simulink model "Esercitazione__2"  (R2023b)
settings: Solver=VariableStepAuto  StartTime=0.0  StopTime=10.0  RelTol=1e-3
values from neighbouring files (symbols this model uses):
  CLi = CLvec(j)    [es2.m]    (also in es2_deflussaggio.m)
  Vaprime = Vavec(i)    [es2.m]    (also in es2_deflussaggio.m = 1)
  Vfprime = 1    [es2.m]    (also in es2_deflussaggio.m = bvec(i))
undefined symbols (not defined in the file or in its folder): kteta, kw, taua, Te, Tm, Tteta
settings Model: Creator=marco  LastModifiedBy=39327

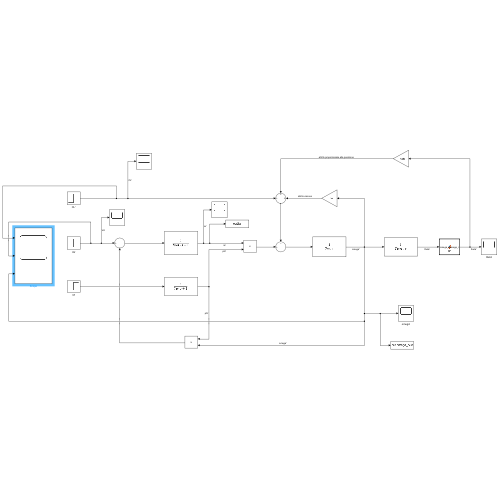
[thumbnail: Simulink's stored preview of the top-level diagram]
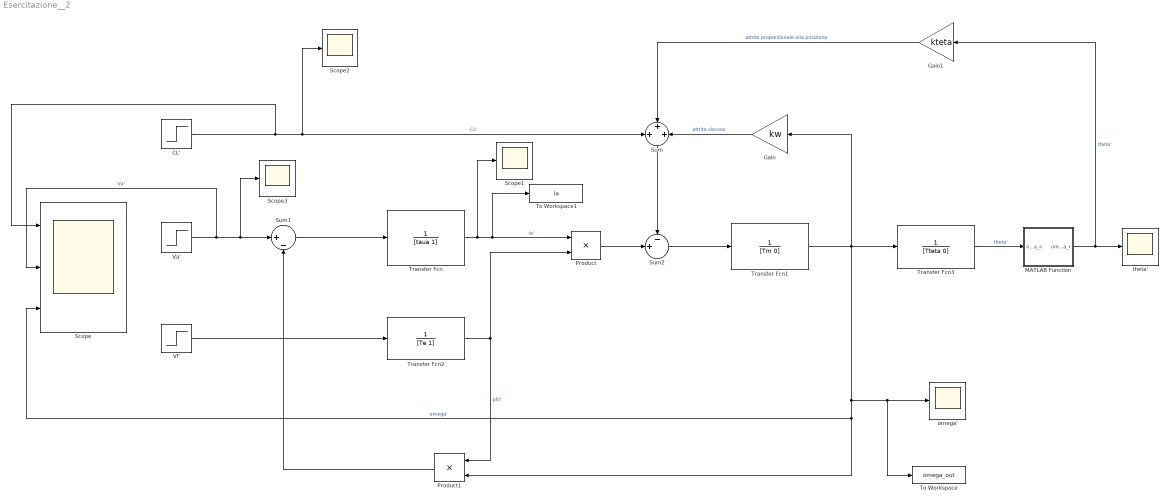
== system Esercitazione__2 ==
  CL' : Step  Time=3  After=CLi  SampleTime=0
  Gain : Gain  Gain=kw
  Gain1 : Gain  Gain=kteta
  MATLAB Function : MATLAB Function  TreatAsAtomicUnit=on
  Product : Product
  Product1 : Product
  Scope : Scope  NumInputPorts=3
  Scope1 : Scope
  Scope2 : Scope
  Scope3 : Scope
  Sum : Sum  Inputs=+++
  Sum1 : Sum  Inputs=|+-
  Sum2 : Sum  Inputs=-+|
  To Workspace : ToWorkspace  VariableName=omega_out  SaveFormat=Structure With Time  SampleTime=-1
  To Workspace1 : ToWorkspace  VariableName=ia  SaveFormat=Structure With Time  SampleTime=-1
  Transfer Fcn : TransferFcn  Denominator=[taua 1]
  Transfer Fcn1 : TransferFcn  Denominator=[Tm 0]
  Transfer Fcn2 : TransferFcn  Denominator=[Te 1]
  Transfer Fcn3 : TransferFcn  Denominator=[Tteta 0]
  Va' : Step  After=Vaprime  SampleTime=0
  Vf' : Step  Time=0  After=Vfprime  SampleTime=0
  omega' : Scope
  theta' : Scope
  wires:
  Va'/1 -> Scope/2, Scope3/1, Sum1/1  "Va'"
  Sum1/1 -> Transfer Fcn/1
  Vf'/1 -> Transfer Fcn2/1
  Transfer Fcn2/1 -> Product1/1, Product/2  "phi'"
  Product/1 -> Sum2/2
  Sum2/1 -> Transfer Fcn1/1
  Sum/1 -> Sum2/1
  CL'/1 -> Scope/1, Sum/1, Scope2/1  "CL'"
  Gain/1 -> Sum/3  "attrito viscoso"
  Transfer Fcn1/1 -> To Workspace/1, omega'/1, Scope/3, Product1/2, Gain/1, Transfer Fcn3/1  "omega'"
  Transfer Fcn3/1 -> MATLAB Function/1(omega_n)  "theta'"
  MATLAB Function/1(omega_r) -> Gain1/1, theta'/1  "theta'"
  Gain1/1 -> Sum/2  "attrito proporzionale alla posizione"
  Product1/1 -> Sum1/2
  Transfer Fcn/1 -> Scope1/1, To Workspace1/1, Product/1  "ia'"

== matlab function Esercitazione__2/MATLAB Function ==
  data: omega_n input; omega_r output
function omega_r = fcn(omega_n)
omega_r = rem(omega_n,2*pi);
end
